simulink model "zxy2_1"  (R2017b)
settings: Solver=VariableStepAuto  StartTime=0.0  StopTime=10.0  RelTol=1e-3
settings Model: Creator=zxy19  LastModifiedBy=zxy19

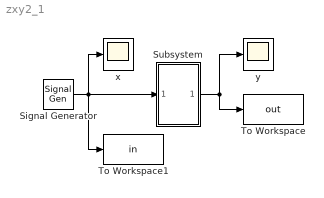
== system zxy2_1 ==
  Signal Generator : SignalGenerator  WaveForm=sawtooth  Amplitude=5  Frequency=0.25
  Subsystem : Subsystem  mask{a=1, b=1, c=1}
  To Workspace : ToWorkspace  VariableName=out  SaveFormat=Timeseries  SampleTime=-1
  To Workspace1 : ToWorkspace  VariableName=in  SaveFormat=Timeseries  SampleTime=-1
  "x " : Scope
  y : Scope
  wires:
  Signal Generator/1 -> "x "/1, To Workspace1/1, Subsystem/1(In1)
  Subsystem/1(Out1) -> y/1, To Workspace/1

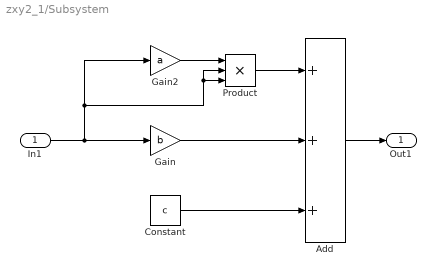
== system zxy2_1/Subsystem ==
  In1 : Inport
  Add : Sum  Inputs=+++
  Constant : Constant  Value=c
  Gain : Gain  Gain=b
  Gain2 : Gain  Gain=a
  Product : Product  Inputs=3
  Out1 : Outport
  wires:
  In1/1 -> Gain2/1, Product/3, Product/2, Gain/1
  Gain/1 -> Add/2
  Product/1 -> Add/1
  Gain2/1 -> Product/1
  Constant/1 -> Add/3
  Add/1 -> Out1/1
